simulink library "xrbsDSP_r4"  (Simulink 7.1)
undefined symbols (not defined in the file or in its folder): mem
libraries: xbsIndex_r4 x330
(part 1 of 5)
settings Model: Creator=singhj  LastModifiedBy=sysgengroup

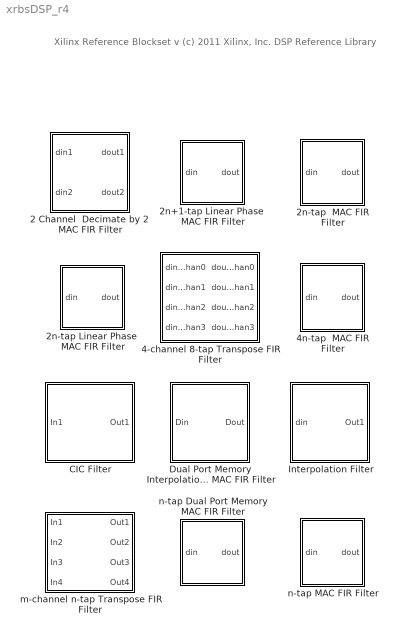
== system xrbsDSP_r4 ==
  note: Xilinx Reference Blockset v
      | (c) 2011 Xilinx, Inc.
      |
      | DSP Reference Library
  2 Channel  Decimate by 2  MAC FIR Filter : Subsystem  mask(n tap 2 Channel Decimate by 2 MAC FIR Filter){bit_width=18, bin_pt=16, coef1=fir1(60,.1), coef2=fir1(60,.3), coef_bit_width=18, coef_bin_pt=18, Ts=1}
      mask prompts: bit_width "Data Input Bit Width"; bin_pt "Data Input Binary Point"; coef1 "Coefficient Vector (Ch.1)"; coef2 "Coefficient Vector (Ch.2)"; coef_bit_width "Number of Bits per Coefficient"; coef_bin_pt "Binary Point per Coefficient"; Ts "Sample Period"
      mask help:
      | This is a n tap 2 Channel Filter decimate by 2 MAC Based FIR Filter.
      |
      |  - The Data Input bit width should be the same for both ports.
      |  - The number of Coefficients must be the same for both channels.
      |  - Pad coefficients with zeros if necessary.
      mask init:
      | %make sure there are an even number of coefficients
      | even_test1 = length(coef1)/2 - floor(length(coef1)/2);
      | if (even_test1 > 0)
      | 	coef1 = [coef1(:)' 0];
      | end
      | 
      | even_test2 = length(coef2)/2 - floor(length(coef2)/2);
      | if (even_test2 > 0)
      | 	coef2 = [coef2(:)' 0];
      | end
      | 
      | coef = 0;
      | j = 0;
      | 
      | for i = 1:2:length(coef1)
      | 
      | 	j = j+1;
      | 	coef(j) = coef1(i);
      | 
      | end
      | 
      | for i = 1:2:length(coef2)
      | 
      | 	j = j+1;
      | 	coef(j) = coef2(i);
      | 
      | end
      | 
      | for i = 2:2:length(coef1)
      | 
      | 	j = j+1;
      | 	coef(j) = coef1(i);
      | 
      | end
      | 
      | for i = 2:2:length(coef2)
      | 
      | 	j = j+1;
      | 	coef(j) = coef2(i);
      | 
      | end
      | 
      | %calculate the largest phase filter coefficient sum
      | 
      | %work in integers firstly
      | coef_int = coef*2^coef_bin_pt;
      | %Sum the coefficients
      | coef_sum1 = sum(abs(coef_int(1:length(coef_int)/4)));
      | coef_sum2 = sum(abs(coef_int(length(coef_int)/2+1:3*length(coef_int)/4)));
      | 
      | if coef_sum1 >= coef_sum2
      | 	coef_sum = coef_sum1;
      | else
      | 	coef_sum = coef_sum2;
      | end
      | 
      | %calculate the 2nd accumalator output width. Accomdates for poor coefficients
      | accum2_temp = ceil(log2(coef_sum*(2^(bit_width-1))))+1;
      | if accum2_temp < (bit_width+coef_bit_width)
      | 	accum2_bit_width = bit_width+coef_bit_width;
      | else
      | 	accum2_bit_width = accum2_temp;
      | end
      | 
      | %Graphic display
      | [bg,fg] = xlcmap('XBlock',0);
      | iPos = get_param(gcb,'Position');
      | iWidth=iPos(3)-iPos(1); iHeight=iPos(4)-iPos(2);
      | iCx=iWidth/2;
      | iCy=iHeight/2;
      | [logoX, logoY] = xlogo(iPos);
      mask Help: eval('');xlDoc('-book','sysgen','-topic','x2_Channel__Decimate_by_2__MAC_FIR_Filter');
      mask Display:
      | patch([0 iWidth iWidth 0],[0 0 iHeight iHeight] , bg);
      | patch(logoX,logoY , fg);
      | plot([0 0 iWidth iWidth 0], [0 iHeight iHeight 0 0]);
      | 
      | disp(sprintf('%d tap\nMAC FIR',length(coef)/2) )
      | 
      | port_label ('output',1,'yn0')
      | port_label ('output',2,'yn1')
      | port_label ('input',1,'xn0')
      | port_label ('input',2,'xn1')
  2n+1-tap Linear Phase  MAC FIR Filter : Subsystem  mask(2n+1-tap Linear Phase MAC FIR Filter){coef=fir1(32,.5), coef_n_bits=12, coef_bin_pt=11, smpl_n_bits=12, smpl_bin_pt=8, smpl_period=1}
      mask prompts: coef "Coefficients"; coef_n_bits "Number of Bits per Coefficient"; coef_bin_pt "Binary Point for Coefficient"; smpl_n_bits "Number of Bits per Input Sample"; smpl_bin_pt "Binary Point for Input Samples"; smpl_period "Input Sample Period"
      mask help: Linear phase MAC-based FIR filter with 2*n+1 coefficients. Design exploits odd coefficient symmetry.
      mask init:
      | dstr = sprintf('%d tap',length(coef));
      | 
      | [bg,fg] = xlcmap('XBlock',0);
      | iPos = get_param(gcb,'Position');
      | iWidth=iPos(3)-iPos(1); iHeight=iPos(4)-iPos(2);
      | iCx=iWidth/2;
      | iCy=iHeight/2;
      | [logoX, logoY] = xlogo(iPos);
      mask Help: eval('');xlDoc('-book','sysgen','-topic','x2n_1_tap_Linear_Phase__MAC_FIR_Filter');
      mask Display:
      | patch([0 iWidth iWidth 0],[0 0 iHeight iHeight] , bg);
      | patch(logoX,logoY, fg);
      | text(iCx/1.8,iCy+2,dstr);
      | text(iCx/2.0-4,iCy-10,'MAC FIR');
      | plot([0 0 iWidth iWidth 0], [0 iHeight iHeight 0 0]);
  2n-tap  MAC FIR Filter : Subsystem  mask(2n-tap MAC FIR Filter){coef=fir1(31,.5), coef_n_bits=12, coef_bin_pt=11, smpl_n_bits=12, smpl_bin_pt=8, smpl_period=1}
      mask prompts: coef "Coefficients"; coef_n_bits "Number of Bits per Coefficient"; coef_bin_pt "Binary Point for Coefficient"; smpl_n_bits "Number of Bits per Input Sample"; smpl_bin_pt "Binary Point for Input Samples"; smpl_period "Input Sample Period"
      mask help: MAC-based FIR filter with 2*n coefficients. Number of coefficients must be divisible by 2.
      mask init: same as xrbsDSP_r4/2n+1-tap Linear Phase  MAC FIR Filter
      mask Help: eval('');xlDoc('-book','sysgen','-topic','x2n_tap__MAC_FIR_Filter');
      mask Display:
      | patch([0 iWidth iWidth 0],[0 0 iHeight iHeight] , bg);
      | patch(logoX,logoY, fg);
      | text(iCx/1.8,iCy+2,dstr);
      | text(iCx/2.0-4,iCy-10,'MAC FIR');
      | plot([0 0 iWidth iWidth 0], [0 iHeight iHeight 0 0]);
  2n-tap Linear Phase  MAC FIR Filter : Subsystem  mask(2n-tap Linear Phase MAC FIR Filter){coef=fir1(31,.5), coef_n_bits=12, coef_bin_pt=11, smpl_n_bits=12, smpl_bin_pt=8, smpl_period=1}
      mask prompts: coef "Coefficients"; coef_n_bits "Number of Bits per Coefficient"; coef_bin_pt "Binary Point for Coefficient"; smpl_n_bits "Number of Bits per Input Sample"; smpl_bin_pt "Binary Point for Input Samples"; smpl_period "Input Sample Period"
      mask help: Linear phase MAC-based FIR filter with 2*n coefficients. Design exploits even coefficient symmetry.
      mask init: same as xrbsDSP_r4/2n+1-tap Linear Phase  MAC FIR Filter
      mask Help: eval('');xlDoc('-book','sysgen','-topic','x2n_tap_Linear_Phase__MAC_FIR_Filter');
      mask Display:
      | patch([0 iWidth iWidth 0],[0 0 iHeight iHeight] , bg);
      | patch(logoX,logoY, fg);
      | text(iCx/1.8,iCy+2,dstr);
      | text(iCx/2.0-4,iCy-10,'MAC FIR');
      | plot([0 0 iWidth iWidth 0], [0 iHeight iHeight 0 0]);
  4-channel 8-tap Transpose FIR Filter : Subsystem  mask(4-channel 8-tap Transpose FIR Filter){coef=fir1(7,.5), coef_n_bits=12, coef_bin_pt=11, smpl_n_bits=12, smpl_bin_pt=8, smpl_period=1}
      mask prompts: coef "Coefficients"; coef_n_bits "Number of Bits per Coefficient"; coef_bin_pt "Binary Point for Coefficient"; smpl_n_bits "Number of Bits per Input Sample"; smpl_bin_pt "Binary Point for Input Samples"; smpl_period "Input Sample Period"
      mask help: 4-channel 8-tap transpose FIR filter implemented using Virtex-II dedicated multipliers.
      mask init:
      | [bg,fg] = xlcmap('XBlock',0);
      | iPos = get_param(gcb,'Position');
      | iWidth=iPos(3)-iPos(1); iHeight=iPos(4)-iPos(2);
      | iCx=iWidth/2;
      | iCy=iHeight/2;
      | [logoX, logoY] = xlogo(iPos);
      mask Help: eval('');xlDoc('-book','sysgen','-topic','x4_channel_8_tap_Transpose_FIR_Filter');
      mask Display:
      | patch([0 iWidth iWidth 0],[0 0 iHeight iHeight] , bg);
      | patch(logoX,logoY, fg);
      | port_label('input',1,'xn0');
      | port_label('input',2,'xn1');
      | port_label('input',3,'xn2');
      | port_label('input',4,'xn3');
      | port_label('output',1,'yn0');
      | port_label('output',2,'yn1');
      | port_label('output',3,'yn2');
      | port_label('output',4,'yn3');
      | plot([0 0 iWidth iWidth 0], [0 iHeight iHeight 0 0]);
      | 
      | disp('8 Tap\n4 Channel\nTranspose\nFIR Filter')
  4n-tap  MAC FIR Filter : Subsystem  mask(4n-tap MAC FIR Filter){coef=fir1(63,.5), coef_n_bits=12, coef_bin_pt=11, smpl_n_bits=12, smpl_bin_pt=8, smpl_period=1}
      mask prompts: coef "Coefficients"; coef_n_bits "Number of Bits per Coefficient"; coef_bin_pt "Binary Point for Coefficient"; smpl_n_bits "Number of Bits per Input Sample"; smpl_bin_pt "Binary Point for Input Samples"; smpl_period "Input Sample Period"
      mask help: MAC-based FIR filter with 4*n coefficients. Number of coefficients must be divisible by 4.
      mask init:
      | dstr = sprintf('%d tap',length(coef));
      | 
      | [bg,fg] = xlcmap('XBlock',0);
      | iPos = get_param(gcb,'Position');
      | iWidth=iPos(3)-iPos(1); iHeight=iPos(4)-iPos(2);
      | iCx=iWidth/2;
      | iCy=iHeight/2;
      | [logoX, logoY] = xlogo(iPos);
      mask Help: eval('');xlDoc('-book','sysgen','-topic','x4n_tap__MAC_FIR_Filter');
      mask Display:
      | patch([0 iWidth iWidth 0],[0 0 iHeight iHeight] , bg);
      | patch(logoX,logoY, fg);
      | text(iCx/1.8,iCy+2,dstr);
      | text(iCx/2.0-4,iCy-10,'MAC FIR');
      | plot([0 0 iWidth iWidth 0], [0 iHeight iHeight 0 0]);
  CIC Filter : Subsystem  mask(CIC Filter){input_bitwidth=18, input_binpt=16, filter_type=Decimator, rate_change=48, stages=3, m=1, pipeline=on}
      mask prompts: input_bitwidth "Input Bit Width"; input_binpt "Input Binary Point"; filter_type "Filter Type"; rate_change "Sample Rate Change"; stages "Number of Stages"; m "Differential Delay"; pipeline "Pipeline Differentiators"
      mask help: Cascaded Integrated Comb (CIC) Filter
      mask init:
      | % CIC Single Channel v1.0
      | % Set Block Logo
      | sav_gcb=gcb;
      | [bg,fg] = xlcmap('XBlock',0);
      | iPos = get_param(sav_gcb,'Position');
      | iWidth=iPos(3)-iPos(1); iHeight=iPos(4)-iPos(2);
      | iCx=iWidth/2;
      | iCy=iHeight/2;
      | [logoX, logoY] = xlogo(iPos);
      | 
      | % Determine previous filter type and number of stages
      | prev_stages_list = find_system(sav_gcb, 'lookUnderMasks', 'all', 'FollowLinks', 'on', 'Regexp', 'on', 'Name', '^Integrator*'); %this is a cell array
      | prev_stages = length(prev_stages_list);
      | 
      | prev_filter_list = find_system(sav_gcb, 'lookUnderMasks', 'all', 'FollowLinks', 'on', 'Regexp', 'on', 'Name', '^Up Sample*'); %this is a cell array
      | if (isempty(prev_filter_list))
      |     prev_filter_list = find_system(sav_gcb, 'lookUnderMasks', 'all', 'FollowLinks', 'on', 'Regexp', 'on', 'Name', '^Down Sample*'); %this is a cell array
      |     if (isempty(prev_filter_list))
      |         errordlg('Previous Filter Type could not be determined')
      |     else
      |         prev_filter_type = 2;
      |     end
      | else
      |     prev_filter_type = 1;
      | end
      |   
      |   
      | % Print label on the block
      | if(filter_type == 2)
      |    cic_str = sprintf('%d-Stage\n CIC\n%d:1 Decimator',stages, rate_change);
      | else
      |    cic_str = sprintf('%d-Stage\n CIC\n1:%d Interpolator',stages, rate_change);	
      | end
      | 
      | % Make sure the entered values for stages and channels are positive integers
      | nstages = round(sum(abs(stages)));
      | 
      | % issue an error if the number of stages entered is zero
      | if (nstages == 0)
      | 	nstages = prev_stages;
      | 	errordlg('Number of Stages must be more than zero')
      | end
      | 
      | if (nstages == prev_stages) & (filter_type == prev_filter_type)
      |     return
      | end
      | 
      | if(filter_type == 2) % Decimator
      |    if (prev_filter_type == 1) % was interpolator so turn to decimator
      |        for i= 2:prev_stages,
      | 	      delete_line(sav_gcb, ['Integrator' int2str(i-1) '/' int2str(1)], ['Integrator' int2str(i) '/' int2str(1)]);
      | 	      delete_line(sav_gcb, ['Differentiator' int2str(i-1) '/' int2str(1)], ['Differentiator' int2str(i) '/' int2str(1)]);
      |        end
      | 
      |        % disconnect the last blocks in the two sections
      |        delete_line(sav_gcb, ['Differentiator' int2str(prev_stages) '/' int2str(1)], ['Up Sample/1']);
      |        delete_line(sav_gcb, ['Integrator' int2str(prev_stages) '/' int2str(1)], 'Out1/1');
      | 	
      | 	   % delete the line from the Up sampler to the Integrator
      | 	   delete_line(sav_gcb, 'Up Sample/1', 'Integrator1/1'); 
      | 	   delete_line(sav_gcb, 'In1/1', 'Differentiator1/1'); 
      | 	   
      | 	   % Delete the Up Sampler and then replace with an Down Sampler
      | 	   pup = get_param([sav_gcb '/Up Sample'], 'position');
      | 	   delete_block([sav_gcb '/Up Sample']);
      | 	   load_system('xbsIndex_r4');
      | 	   add_block('xbsIndex_r4/Down Sample', [sav_gcb '/Down Sample'], 'sample_ratio', 'rate_change','sample_phase', 'First Value of Frame', 'position', [pup(1), pup(2), pup(3),pup(4)]);
      | 	   
      | 	   % Switch the Integrators and Decimators around
      | 	   for i=1:prev_stages,
      | 		   tempi = get_param([sav_gcb '/Integrator' int2str(i)], 'position');
      | 	       tempd = get_param([sav_gcb '/Differentiator' int2str(i)], 'position');
      | 		   set_param([sav_gcb '/Differentiator' int2str(i)], 'position', [tempi(1), tempi(2), tempi(3), tempi(4)], 'output_bitwidth', 'ceil(stages*log2(rate_change*m) + input_bitwidth)');
      | 		   set_param([sav_gcb '/Integrator' int2str(i)], 'position', [tempd(1), tempd(2), tempd(3), tempd(4)]);
      | 	   end
      | 	   	   	
      | 	   % add back in the lines
      |        add_line(sav_gcb, 'In1/1', 'Integrator1/1', 'autorouting', 'on');
      | 	   add_line(sav_gcb, ['Integrator' int2str(prev_stages) '/1'], 'Down Sample/1', 'autorouting', 'on');
      | 	   add_line(sav_gcb, 'Down Sample/1', 'Differentiator1/1', 'autorouting', 'on');
      | 	   add_line(sav_gcb, ['Differentiator' int2str(prev_stages) '/1'], 'Out1/1', 'autorouting', 'on');
      | 	   for i= 2:prev_stages,
      |           add_line(sav_gcb, ['Integrator' int2str(i-1) '/1'], ['Integrator' int2str(i) '/' int2str(1)], 'autorouting', 'on');
      |           add_line(sav_gcb, ['Differentiator' int2str(i-1) '/1'], ['Differentiator' int2str(i) '/' int2str(1)], 'autorouting', 'on');
      | 	   end
      | 		
      |        %Set the Output bit widths of Differentiator and Integrator stages
      |        set_param([sav_gcb '/Differentiator1'], 'output_bitwidth', 'ceil(stages*log2(rate_change*m) + input_bitwidth)');
      | 	   	   %Set the Output bit width of Integrator stages
      | 	   %Calculate the Interpolator Integrator Output Bit Growth
      |        for i= 1:prev_stages,
      | 			 j = nstages+i;
      | 	         set_param([sav_gcb '/Integrator' int2str(i)], 'output_bitwidth', 'ceil(stages*log2(rate_change*m) + input_bitwidth)');
      |              set_param([sav_gcb '/Differentiator' int2str(i)], 'output_bitwidth', 'ceil(stages*log2(rate_change*m) + input_bitwidth)');
      | 	   end
      | 	   
      |    end
      |    
      |    if (nstages ~= prev_stages)
      |     
      |        % disconnect all the wires from all the blocks
      |        for i= 2:prev_stages,
      | 	      delete_line(sav_gcb, ['Integrator' int2str(i-1) '/' int2str(1)], ['Integrator' int2str(i) '/' int2str(1)]);
      | 	      delete_line(sav_gcb, ['Differentiator' int2str(i-1) '/' int2str(1)], ['Differentiator' int2str(i) '/' int2str(1)]);
      |        end
      | 
      |        % disconnect the last blocks in the two sections
      |        delete_line(sav_gcb, ['Integrator' int2str(prev_stages) '/' int2str(1)], ['Down Sample/1']);
      |        delete_line(sav_gcb, ['Differentiator' int2str(prev_stages) '/' int2str(1)], 'Out1/1');
      | 	
      | 	   % delete the line from the down sampler to the differentiator
      | 	   delete_line(sav_gcb, 'Down Sample/1', 'Differentiator1/1');
      | 	
      | 	   % Remove all the blocks except the first one (as we always will have one)
      |        for i=2:prev_stages,
      | 		  delete_block([sav_gcb '/Differentiator' int2str(i)]);
      | 	      delete_block([sav_gcb '/Integrator' int2str(i)]);
      |        end
      | 	   
      | 	   %Set the Output bit width of Differentiator stages
      |        set_param([sav_gcb '/Differentiator1'], 'output_bitwidth', 'ceil(stages*log2(rate_change*m) + input_bitwidth)');
      | 	   
      | 	   % collect data on the position of existing blocks
      | 	   pi = get_param([sav_gcb '/Integrator1'], 'position');
      | 	   pd = get_param([sav_gcb '/Differentiator1'], 'position');
      | 	   set_param([sav_gcb '/Differentiator1'], 'position', [pi(1)+(nstages+1)*80, pd(2), pi(3)+(nstages+1)*80, pd(4)]);
      | 	   pd = get_param([sav_gcb '/Differentiator1'], 'position');
      | 	
      | 	   % move the current blocks to accomadate for new blocks to be added 
      | 	   pds = get_param([sav_gcb '/Down Sample'], 'position');
      | 	   set_param([sav_gcb '/Down Sample'], 'position', [pi(1)+(nstages)*80, pds(2), pi(3)+(nstages)*80, pds(4)]);
      | 	   
      | 	   po = get_param([sav_gcb '/Out1'], 'position');
      | 	   set_param([sav_gcb '/Out1'], 'position', [pd(1)+(nstages+1)*80, po(2), pd(1)+(po(3)-po(1))+(nstages+1)*80, po(4)]);	
      | 	
      | 	   % add back in the line between the Down Sampler and the 1st Differentiator
      |        add_line(sav_gcb, 'Down Sample/1', ['Differentiator1/' int2str(1)], 'autorouting', 'on');
      | 
      | 	   % Only add blocks if more than one stage is required
      | 	   if (nstages ~= 1)
      | 		
      | 	       % Add in a copy of the first block to make up the required number of stages
      |            for i=2:nstages,
      |                add_block([sav_gcb '/Integrator1'], [sav_gcb '/Integrator' int2str(i)], 'position', [pi(1)+(i-1)*80, pi(2), pi(3)+(i-1)*80, pi(4)]);
      | 		       add_block([sav_gcb '/Differentiator1'], [sav_gcb '/Differentiator' int2str(i)], 'position', [pd(1)+(i-1)*80, pd(2), pd(3)+(i-1)*80, pd(4)]);
      | 	       end
      | 		
      | 	       % Connect up the wires to each block use autorouting
      |            for i= 2:nstages,
      |  		       add_line(sav_gcb, ['Integrator' int2str(i-1) '/' int2str(1)], ['Integrator' int2str(i) '/' int2str(1)], 'autorouting', 'on');
      | 	           add_line(sav_gcb, ['Differentiator' int2str(i-1) '/' int2str(1)], ['Differentiator' int2str(i) '/' int2str(1)], 'autorouting', 'on');
      |            end
      | 	    end
      | 	       % Connect the last blocks in the two sections
      |            add_line(sav_gcb, ['Integrator' int2str(nstages) '/' int2str(1)], ['Down Sample/1'], 'autorouting', 'on');
      |            add_line(sav_gcb, ['Differentiator' int2str(nstages) '/' int2str(1)], ['Out1/1'], 'autorouting', 'on');
      |    end
      | 
      | else % Interpolator
      |    
      | 	
      | 	if (prev_filter_type == 2) % was decimator so turn to interpolator
      | 	
      | 	  % disconnect all the wires from all the blocks
      |        for i= 2:prev_stages,
      | 	      delete_line(sav_gcb, ['Integrator' int2str(i-1) '/' int2str(1)], ['Integrator' int2str(i) '/' int2str(1)]);
      | 	      delete_line(sav_gcb, ['Differentiator' int2str(i-1) '/' int2str(1)], ['Differentiator' int2str(i) '/' int2str(1)]);
      |        end
      | 
      |        % disconnect the last blocks in the two sections
      |        delete_line(sav_gcb, ['Integrator' int2str(prev_stages) '/' int2str(1)], ['Down Sample/1']);
      |        delete_line(sav_gcb, ['Differentiator' int2str(prev_stages) '/' int2str(1)], 'Out1/1');
      | 	
      | 	   % delete the line from the down sampler to the Differentiator
      | 	   delete_line(sav_gcb, 'Down Sample/1', 'Differentiator1/1'); 
      | 	   delete_line(sav_gcb, 'In1/1', 'Integrator1/1'); 
      | 	   
      | 	   % Delete the Down Sampler and then replace with a Up Sampler
      | 	   pdwn = get_param([sav_gcb '/Down Sample'], 'position');
      | 	   delete_block([sav_gcb '/Down Sample']);
      | 	   load_system('xbsIndex_r4');
      | 	   add_block('xbsIndex_r4/Up Sample', [sav_gcb '/Up Sample'], 'sample_ratio', 'rate_change', 'position', [pdwn(1), pdwn(2), pdwn(3), pdwn(4)]);
      | 	   
      | 	   % Switch the Integrators and Decimators around
      | 	   for i=1:prev_stages,
      | 		   tempi = get_param([sav_gcb '/Integrator' int2str(i)], 'position');
      | 	       tempd = get_param([sav_gcb '/Differentiator' int2str(i)], 'position');
      | 		   set_param([sav_gcb '/Differentiator' int2str(i)], 'position', [tempi(1), tempi(2), tempi(3), tempi(4)], 'output_bitwidth', [int2str(i) '+ input_bitwidth']);
      | 		   set_param([sav_gcb '/Integrator' int2str(i)], 'position', [tempd(1), tempd(2), tempd(3), tempd(4)]);
      | 	   end
      | 	   	   	
      | 	   % add back in the lines
      |        add_line(sav_gcb, 'In1/1', 'Differentiator1/1', 'autorouting', 'on');
      | 	   add_line(sav_gcb, ['Differentiator' int2str(prev_stages) '/1'], 'Up Sample/1', 'autorouting', 'on');
      | 	   add_line(sav_gcb, 'Up Sample/1', 'Integrator1/1', 'autorouting', 'on');
      | 	   add_line(sav_gcb, ['Integrator' int2str(prev_stages) '/1'], 'Out1/1', 'autorouting', 'on');
      | 	   for i= 2:prev_stages,
      |           add_line(sav_gcb, ['Integrator' int2str(i-1) '/1'], ['Integrator' int2str(i) '/1'], 'autorouting', 'on');
      |           add_line(sav_gcb, ['Differentiator' int2str(i-1) '/1'], ['Differentiator' int2str(i) '/1'], 'autorouting', 'on');
      | 	   end
      | 	   
      | 	   %Set the Output bit width of Integrator stages
      | 	   %Calculate the Interpolator Integrator Output Bit Growth
      |        for i= 1:prev_stages,
      | 			 j = nstages+i;
      | 	         set_param([sav_gcb '/Integrator' int2str(i)], 'output_bitwidth', ['ceil(log2(2^(2*stages-' int2str(j) ')*(rate_change*m)^(' int2str(j) '-stages)) + input_bitwidth)']);
      | 	   end
      | 		
      |    end
      |    
      | 	
      | 	if (nstages ~= prev_stages)
      |     
      |        % disconnect all the wires from all the blocks
      |        for i= 2:prev_stages,
      | 	      delete_line(sav_gcb, ['Integrator' int2str(i-1) '/' int2str(1)], ['Integrator' int2str(i) '/' int2str(1)]);
      | 	      delete_line(sav_gcb, ['Differentiator' int2str(i-1) '/' int2str(1)], ['Differentiator' int2str(i) '/' int2str(1)]);
      |        end
      | 
      |        % disconnect the last blocks in the two sections
      |        delete_line(sav_gcb, ['Differentiator' int2str(prev_stages) '/' int2str(1)], ['Up Sample/1']);
      |        delete_line(sav_gcb, ['Integrator' int2str(prev_stages) '/' int2str(1)], 'Out1/1');
      |        
      | 	
      | 	   % delete the line from the Up sampler to the Integrator1 for movement later
      | 	   delete_line(sav_gcb, 'Up Sample/1', 'Integrator1/1'); 
      | 	
      | 	   % Remove all the blocks except the first one (as we always will have one)
      |        for i=2:prev_stages,
      | 		  delete_block([sav_gcb '/Differentiator' int2str(i)]);
      | 	      delete_block([sav_gcb '/Integrator' int2str(i)]);
      |        end
      | 	
      | 	   %Set the Output bit width of first Differentiator stage (other are set as copies of this block)
      |        set_param([sav_gcb '/Differentiator1'], 'output_bitwidth', '1 + input_bitwidth');
      | 	   
      | 	   % collect data on the position of existing blocks
      | 	   pi = get_param([sav_gcb '/Integrator1'], 'position');
      | 	   pd = get_param([sav_gcb '/Differentiator1'], 'position');
      | 	   set_param([sav_gcb '/Integrator1'], 'position', [pd(1)+(nstages+1)*80, pi(2), pd(3)+(nstages+1)*80, pi(4)]);
      | 	   pi = get_param([sav_gcb '/Integrator1'], 'position');
      | 	
      | 	   % move the current blocks to accomadate for new blocks to be added 
      | 	   pus = get_param([sav_gcb '/Up Sample'], 'position');
      | 	   set_param([sav_gcb '/Up Sample'], 'position', [pd(1)+(nstages)*80, pus(2), pd(3)+(nstages)*80, pus(4)]);
      | 	
      | 	   po = get_param([sav_gcb '/Out1'], 'position');
      |        set_param([sav_gcb '/Out1'], 'position', [pi(1)+(nstages+1)*80, po(2), pi(1)+(po(3)-po(1))+(nstages+1)*80, po(4)]);	
      |       
      | 	
      | 	   % add back in the line between the Up Sampler and the 1st Integrator1
      | 	   add_line(sav_gcb, 'Up Sample/1', 'Integrator1/1', 'autorouting', 'on');
      | 	   
      | 	   % Only add blocks if more than one stage is required
      | 	   if (nstages ~= 1)
      | 		
      | 	       % Add in a copy of the first block to make up the required number of stages
      |            for i=2:nstages,
      |                add_block([sav_gcb '/Integrator1'], [sav_gcb '/Integrator' int2str(i)], 'position', [pi(1)+(i-1)*80, pi(2), pi(3)+(i-1)*80, pi(4)]);
      | 		       add_block([sav_gcb '/Differentiator1'], [sav_gcb '/Differentiator' int2str(i)], 'position', [pd(1)+(i-1)*80, pd(2), pd(3)+(i-1)*80, pd(4)], 'output_bitwidth', [int2str(i) '+ input_bitwidth']);
      | 	       end
      | 		
      | 	       % Connect up the wires to each block use autorouting
      |            for i= 2:nstages,
      |  		       add_line(sav_gcb, ['Integrator' int2str(i-1) '/' int2str(1)], ['Integrator' int2str(i) '/' int2str(1)], 'autorouting', 'on');
      | 	           add_line(sav_gcb, ['Differentiator' int2str(i-1) '/' int2str(1)], ['Differentiator' int2str(i) '/' int2str(1)], 'autorouting', 'on');
      |            end
      | 	    end
      | 	       % Connect the last blocks in the two sections
      |            add_line(sav_gcb, ['Differentiator' int2str(nstages) '/1'], ['Up Sample/1'], 'autorouting', 'on');
      |            add_line(sav_gcb, ['Integrator' int2str(nstages) '/1'], ['Out1/1'], 'autorouting', 'on');
      | 		   
      | 	     %Set the Output bit width of Integrator stages
      | 	     %Calculate the Interpolator Integrator Output Bit Growth
      |           for i= 1:nstages,
      | 			 j = nstages+i;
      | 	         set_param([sav_gcb '/Integrator' int2str(i)], 'output_bitwidth', ['ceil(log2(2^(2*stages-' int2str(j) ')*(rate_change*m)^(' int2str(j) '-stages)) + input_bitwidth)']);
      | 	      end
      |    end
      | 	  
      | end
      | 
      | 
      | % Set the pipelining to ON or OFF on the differentiators
      | if (pipeline == 0)
      | 	for i= 1:nstages
      | 		set_param([sav_gcb '/Differentiator' int2str(i), '/AddSub'], 'latency', '0')
      | 	end
      | else
      | 	for i= 1:nstages
      | 		set_param([sav_gcb '/Differentiator' int2str(i), '/AddSub'], 'latency' ,'1')
      | 	end
      | end
      settings: CopyFcn=set_param(gcb, 'MaskSelfModifiable', 'on', 'LinkStatus', 'none');
      mask Help: eval('');xlDoc('-book','sysgen','-topic','CIC_Filter');
      mask StyleString: edit,edit,popup(Interpolator|Decimator),edit,edit,popup(1|2|3|4),checkbox
      mask Display:
      | patch([0 iWidth iWidth 0],[0 0 iHeight iHeight] , bg);
      | patch(logoX,logoY , fg);
      | plot([0 0 iWidth iWidth 0], [0 iHeight iHeight 0 0]);
      | disp(cic_str)
  Dual Port Memory Interpolation MAC FIR Filter : Subsystem  mask(n-tap Interpolate by N Dual Port Block RAM MAC FIR filter ){bit_width=16, bin_pt=13, coef_raw=fir1(55,0.3), coef_bit_width=18, coef_bin_pt=17, interpolation_rate=1:4, Ts=1}
      mask prompts: bit_width "Data Input Bit Width"; bin_pt "Data input Binary Point"; coef_raw "Coefficients"; coef_bit_width "Number of Bits per Coefficient"; coef_bin_pt "Binary Point Per Coefficient"; interpolation_rate "Interpolation Ratio"; Ts "Sample Period"
      mask help: n-tap Interpolate by N Dual Port Block RAM MAC FIR filter
      mask init:
      | % Interpolation by N Filter v1.0 - 8/9/03
      | %adjust the Interpolation Parameter to give the correct value
      | ir = interpolation_rate + 1;
      | 
      | %calculate how many padding bits are required for BRAM storage
      | if ((coef_bit_width - bit_width)  < 0 )
      | 	data_pad_bits = 0;
      | 	coef_pad_bits = bit_width - coef_bit_width;
      | else
      | 	data_pad_bits = coef_bit_width - bit_width;
      | 	coef_pad_bits = 0;
      | end
      | 
      | %prepare the coefficients for Polyphase structure
      | 
      | no_mults = 1; % for this implementation
      | 
      | %pad the coefficients to be a multiple of the interp_ratio*no_mults
      | multiple_test = round(((ceil(length(coef_raw)/(ir*no_mults))) - (length(coef_raw)/(ir*no_mults))) * (ir*no_mults));
      | if (multiple_test > 0)
      | 	coef_raw = [coef_raw(:)' zeros(1,multiple_test)];
      | end
      | 
      | no_taps = length(coef_raw);
      | phase_taps_per_mult = no_taps/no_mults/ir;
      |     
      | %form phase filters
      | h = zeros(1, no_taps/ir);
      | for p = 0:(ir-1)
      |      h(p+1,:) = coef_raw(p+1: ir :(no_taps-ir+p+1));
      | end
      | 
      | %put the phase filters into one memory
      | coef = h(1,:);
      | for p = 2:ir
      | 	coef = [coef h(p,:)];
      | end
      | 
      | %work in integers firstly
      | coef_int = coef*2^coef_bin_pt;
      | %Sum the coefficients
      | coef_sum = sum(abs(coef_int(1:length(coef_int)/4)));
      | 
      | %calculate the accumalator output width. Accomdates for poor coefficients
      | accum_temp = ceil(log2(coef_sum*(2^(bit_width-1))))+1;
      | if accum_temp < (bit_width+coef_bit_width)
      | 	accum_bit_width = bit_width+coef_bit_width;
      | else
      | 	accum_bit_width = accum_temp;
      | end
      | 
      | dstr1 = sprintf('%d tap', no_taps);
      | dstr2 = sprintf('Interpolate');
      | dstr3 = sprintf('by %d', ir);
      | 
      | [bg,fg] = xlcmap('XBlock',0);
      | iPos = get_param(gcb,'Position');
      | iWidth=iPos(3)-iPos(1); iHeight=iPos(4)-iPos(2);
      | iCx=iWidth/2;
      | iCy=iHeight/2;
      | [logoX, logoY] = xlogo(iPos);
      mask Help: eval('');xlDoc('-book','sysgen','-topic','Dual_Port_Memory_Interpolation_MAC_FIR_Filter');
      mask StyleString: edit,edit,edit,edit,edit,popup(1:2|1:3|1:4|1:5|1:6|1:7|1:8|1:9|1:10),edit
      mask Display:
      | patch([0 iWidth iWidth 0],[0 0 iHeight iHeight] , bg);
      | patch(logoX,logoY, fg);
      | text(iCx/1.3,iCy+15,dstr1);
      | text(iCx/2,iCy+2,dstr2);
      | text(iCx/1.3,iCy-9,dstr3);
      | text(iCx/1.5-4,iCy-20,'MAC FIR');
      | plot([0 0 iWidth iWidth 0], [0 iHeight iHeight 0 0]);
  Interpolation Filter : Subsystem  mask(Interpolation Filter){bit_width=8, bin_pt=6, coef=fir1(28,0.3), coef_bit_width=14, coef_bin_pt=14, interp_rate=1:2, Ts=1}
      mask prompts: bit_width "Input Data Bit Width"; bin_pt "Input Data Binary Point"; coef "Coefficients"; coef_bit_width "Number of bits per Coefficient"; coef_bin_pt "Binary Point per Coefficient"; interp_rate "Interpolation Factor"; Ts "Sample Period"
      mask help:
      | n - tap Interpolation MAC FIR filter.
      |
      |  - Support Interpolation rates of 2, 4, and 8.
      |  - 4 Multiplier and 4 Block RAM Architecture
      |  - Slice estimate provided
      |
      | NOTE: The number of coefficients must be divisible by (4*interpolation factor). If not zeros are padded to the coefficients to insure they are.
      |
      | Hardware notes:
      | This filter employs a 4 multiplier architecture to compute the filter. The highest supported sample rate is calculated by the
      | (input sample rate*(number of cofficients/4))
      mask init:
      | %accounts for the pull down GUI value
      | if (interp_rate == 1)
      | 	interp_ratio = 2;
      | elseif (interp_rate == 2)
      | 	interp_ratio = 4;
      | elseif (interp_rate == 3) 	
      | 	interp_ratio = 8;
      | else 	
      | 	interp_ratio = 16;	
      | end
      | 
      | no_mults = 4; % for this implementation
      | 
      | %pad the coefficients to be a multiple of the interp_ratio*no_mults
      | multiple_test = ((ceil(length(coef)/(interp_ratio*no_mults))) - (length(coef)/(interp_ratio*no_mults))) * (interp_ratio*no_mults);
      | if (multiple_test > 0)
      | 	coef = [coef(:)' zeros(1,multiple_test)];
      | end
      | 
      | no_taps = length(coef);
      | phase_taps_per_mult = no_taps/no_mults/interp_ratio;
      |     
      | %form phase filters h(0:3,)
      | h = zeros(1, no_taps/interp_ratio);
      | for p = 0:(interp_ratio-1)
      |      h(p+1,:) = coef(p+1: interp_ratio :(no_taps-interp_ratio+p+1));
      | end
      | 
      | %form DRAM values
      | mem_space = interp_ratio*no_mults*2^(ceil(log2(no_taps/interp_ratio/no_mults)));
      |         
      | z = zeros(1,(mem_space-no_taps)/interp_ratio/no_mults);
      | %mem = zeros(no_mults,(mem_space/no_mults));
      | 
      | for m = 0:(no_mults-1)
      |     for p = 0:(interp_ratio-1)
      | 		i = p*(mem_space/no_mults/interp_ratio)+1:(p+1)*(mem_space/no_mults/interp_ratio);
      |         mem(m+1,i) = [h(p+1,(m*phase_taps_per_mult)+(1:phase_taps_per_mult)), z];
      |     end
      | end
      | 
      | no_phases = interp_ratio;
      | no_phase_taps = no_taps/no_phases;
      | x_SRL_depth = no_phase_taps/no_mults;
      | upsamp_by = x_SRL_depth*no_phases;
      | downsamp_by = upsamp_by/interp_ratio;
      | T_clock = Ts/upsamp_by;
      | bit_growth = 2 + ceil(log2(x_SRL_depth));
      | y_bit_width = bit_width + coef_bit_width + bit_growth;
      | 
      | %slice count calculation
      | % control module
      |     k = ceil(ceil(log2(x_SRL_depth))/2);
      |     p = ceil(ceil(log2(interp_ratio))/2);
      |     k_p_logic = ceil(ceil((2*k + 2*p)/4)/2); %approx # of LUTs
      |     
      |     % synch delay
      |     delay = ceil(ceil(5/16)/2);
      |     
      |     % h DRAM cost
      | 	h = ceil(4*length(mem(1,:))/16/2*coef_bit_width); % for distmem
      |  	h = 0;   %for BRAM
      | 
      | 	% x buffer
      |     x = ceil(4*ceil(x_SRL_depth/16)*bit_width/2);
      |     
      |     % adder tree
      |     stage1 = 2*ceil((bit_width+coef_bit_width+1)/2);
      |     stage2 = ceil((bit_width+coef_bit_width+2)/2);
      |     
      |     % acc stage
      |     acc = ceil(y_bit_width/2);
      |     capture = acc;
      |     
      |     % downsampling
      |     downsample = ceil(y_bit_width/2);
      | 
      | %Display graphic on the block
      | dstr1 = sprintf('%d tap', no_taps);
      | dstr2 = sprintf('Interpolate');
      | dstr3 = sprintf('by %d', interp_ratio);
      | 
      | [bg,fg] = xlcmap('XBlock',0);
      | iPos = get_param(gcb,'Position');
      | iWidth=iPos(3)-iPos(1); iHeight=iPos(4)-iPos(2);
      | iCx=iWidth/2;
      | iCy=iHeight/2;
      | [logoX, logoY] = xlogo(iPos);
      mask Help: eval('');xlDoc('-book','sysgen','-topic','Interpolation_Filter');
      mask StyleString: edit,edit,edit,edit,edit,popup(1:2|1:4|1:8|1:16),edit
      mask Display:
      | patch([0 iWidth iWidth 0],[0 0 iHeight iHeight] , bg);
      | patch(logoX,logoY, fg);
      | text(iCx/1.3,iCy+15,dstr1);
      | text(iCx/2,iCy+2,dstr2);
      | text(iCx/1.3,iCy-9,dstr3);
      | text(iCx/1.5-4,iCy-20,'MAC FIR');
      | plot([0 0 iWidth iWidth 0], [0 iHeight iHeight 0 0]);
  m-channel n-tap Transpose FIR Filter : Subsystem  mask(Transpose Multi Channel FIR Filter){input_bitwidth=12, input_binpt=10, coef_array=fliplr(fir1(13, 0.31)), coef_bitwidth=16, coef_binpt=14, channels=4, tdm_fe=on, tdd_be=on, Ts=1, area2=[0, 0, 0, 0, 0, 0, 0], use_area2=on, prev_ncoef=14, prev_input_channels=4, prev_output_channels=4}
      mask prompts: input_bitwidth "Input Bit Width"; input_binpt "Input Binary Point"; coef_array "Coefficients (specify in reverse order)"; coef_bitwidth "Coefficients Bit Width"; coef_binpt "Coefficients Binary Point"; channels "Number of Channels"; tdm_fe "Time Division Multiplexer Front End"; tdd_be "Time Division DeMultiplexer Back End"; Ts "Input Sample Period"; area2 "FPGA Area [Slices, FFs, BRAMs, LUTs, IOBs, Emb. Mults, TBUFs]"; use_area2 "Use Area Above For Estimation"; prev_ncoef "Previous Coeff Value"; prev_input_channels "Previous Input Channels"; prev_output_channels "Previous Output Channels"
      mask help:
      | This Parametric Multi-Channel Transpose FIR Filter uses a fully parallel architecture with Time Division Multiplexing. The Time Division Multiplexer and Time Division Demux can be selected to be implemented or not. Embedded Multipliers are used for the multipliers.
      |
      | As the number of coefficients change so to does the structure underneath as the model is dynamically built.
      mask init:
      | sav_gcb=gcb;
      | sav_gcbh= gcbh;
      | % Set Block Logo
      | [bg,fg] = xlcmap('XBlock',0);
      | iPos = get_param(sav_gcb,'Position');
      | iWidth=iPos(3)-iPos(1); iHeight=iPos(4)-iPos(2);
      | iCx=iWidth/2;
      | iCy=iHeight/2;
      | [logoX, logoY] = xlogo(iPos);	
      | 
      | % Calculate Coefficient Specific Output Bit Width
      | % Note:  As the input type is not known (signed or unsigned), the
      | % worst case is assumed; hence use of largest unsigned input value
      | % for the given input bitwidth below.
      | magnitudeLargestUnsignedInput = 2^(input_bitwidth);
      | scaledCoefArray = coef_array * (2^coef_binpt);
      | sumOfLargestProducts = sum(scaledCoefArray * magnitudeLargestUnsignedInput);
      | output_bitwidth = ceil(log2(sumOfLargestProducts)) + 1;  % Add one for sign bit.
      | 
      | output_binpt = input_binpt + coef_binpt;
      | if (output_binpt > output_bitwidth)
      | 	output_binpt = output_bitwidth;
      | end
      | 
      | % Print label on the block
      | str = sprintf('%d Tap\n%d Channel\nTranspose\n FIR Filter',length(coef_array), channels);
      | 
      | 
      | % Make sure the entered value for channels is positive integers
      | nchannels = round(sum(abs(channels)));
      | ncoef = length(coef_array);
      | 
      | % How many input or output channels are required
      | if (tdm_fe == 0)
      | 	input_channels = 1;
      | 	% The latency through the TDM block 
      | 	p = 0;
      | else
      | 	input_channels = nchannels;
      | 	% The latency through the TDM block 
      | 	p = 1;
      | end
      | 
      | if (tdd_be == 0)
      | 	output_channels = 1;
      | else
      | 	output_channels = nchannels;
      | end
      | 
      | % Required for naming the port labels. This section creates an array of names for the icon panel to put on the block
      | ports_in = [1:input_channels 1+zeros(1,256-input_channels)];
      | ports_out = [1:output_channels 1+zeros(1,256-output_channels)];
      | 
      | port_inputnames = cell(256, 1);
      | port_outputnames = cell(256, 1);
      | port_inputnames(:,:) = cellstr('xn0');
      | port_outputnames(:,:) = cellstr('yn0');
      | 
      | for i=1:input_channels,
      | 	port_inputnames(i) = cellstr(['xn' int2str(i-1)]);
      | end
      | for i=1:output_channels,
      | 	port_outputnames(i) = cellstr(['yn' int2str(i-1)]);
      | end
      | % Print label on the block
      | m_str = sprintf('%d Tap\n%d Channel\nTranspose\n FIR Filter',length(coef_array), channels);
      | 
      | % Calculate how many channels are currently in the model
      | % pci = find_system([sav_gcb '/TDM'], 'lookUnderMasks', 'all', 'FollowLinks','on','Blocktype', 'Inport'); %this is a cell array
      | % pco = find_system([sav_gcb '/TDD'], 'lookUnderMasks', 'all', 'FollowLinks','on','Blocktype', 'Outport'); %this is a cell array
      | % prev_input_channels = length(pci(:,1));
      | % prev_output_channels = length(pco(:,1));
      | % %calculate how many coefficients currently in the model
      | % c = find_system(sav_gcb, 'lookUnderMasks', 'all', 'FollowLinks','on','masktype', 'MAD Block');
      | % prev_ncoef = length(c(:,1));
      | 
      | %error check for less than two coefficients
      | if (ncoef < 2)
      | 	ncoef = prev_ncoef;
      | 	errordlg('Number of Coefficients must be at least two')
      | end
      | 
      | if (ncoef ~= prev_ncoef)
      |     
      |        % disconnect all the wires from all the blocks
      |        for i= 2:prev_ncoef,
      | 	      delete_line(sav_gcb, ['MAD' int2str(i-1) '/1'], ['MAD' int2str(i) '/2']);
      | 	      delete_line(sav_gcb, ['TDM/1'], ['MAD' int2str(i) '/1']);
      |        end
      | 
      |        % disconnect the last block
      |        delete_line(sav_gcb, ['MAD' int2str(prev_ncoef) '/1'], ['TDD/1']);
      |        for i=1:prev_output_channels,
      | 	       delete_line(sav_gcb, ['TDD/' int2str(i)], ['Out' int2str(i) '/1']); 
      | 	   end
      | 	   
      | 	   % Remove all the blocks except the first two (as we always will have two)
      |        for i=3:prev_ncoef,
      | 		  delete_block([sav_gcb '/MAD' int2str(i)]);
      |        end
      | 	
      | 	   % collect data on the position of existing blocks
      | 	   pmad = get_param([sav_gcb '/MAD2'], 'position');
      | 	 
      | 	   % move the current blocks to accomadate for new blocks to be added 
      | 	   for i=1:prev_output_channels,
      | 	      po = get_param([sav_gcb '/Out' int2str(i)], 'position');
      | 	      set_param([sav_gcb '/Out' int2str(i)], 'position', [pmad(1)+(ncoef)*80, po(2), pmad(1)+(po(3)-po(1))+(ncoef)*80, po(4)]);	
      |        end
      | 	   
      | 	   ptdd = get_param([sav_gcb '/TDD'], 'position');
      | 	   set_param([sav_gcb '/TDD'], 'position', [pmad(1)+(ncoef-1)*80, ptdd(2), pmad(1)+(ptdd(3)-ptdd(1))+(ncoef-1)*80, ptdd(4)]);
      | 	
      | 	   % Only add MAD blocks if more than two taps are required
      | 	   if (ncoef ~= 2)
      | 		
      | 	       % Add in a copy of the first MAD block to make up the required number of coef
      |            for i=3:ncoef,
      |                add_block([sav_gcb '/MAD1'], [sav_gcb '/MAD' int2str(i)], 'position', [pmad(1)+(i-2)*80, pmad(2), pmad(3)+(i-2)*80, pmad(4)], 'coef', ['coef_array(' int2str(i) ')'], 'channels', 'channels');
      | 		   end
      | 		
      | 	       % Connect up the wires to each block use autorouting
      |            for i= 2:ncoef,
      |  		       add_line(sav_gcb, ['MAD' int2str(i-1) '/1'], ['MAD' int2str(i) '/2'], 'autorouting', 'on');
      | 	           add_line(sav_gcb, 'TDM/1', ['MAD' int2str(i) '/1'], 'autorouting', 'on');
      |            end
      | 	   end
      | 	       % Connect the last blocks in the two sections
      |            add_line(sav_gcb, ['MAD' int2str(ncoef) '/1'], ['TDD/1'], 'autorouting', 'on');
      | 		   for i=1:prev_output_channels,
      | 		       add_line(sav_gcb, ['TDD/' int2str(i)], ['Out' int2str(i) '/1'], 'autorouting', 'on');  
      | 		   end
      | end
      | 
      | %%%%%%%%%%%%%%%%%%%%%%%%%%%%%%%%%%%%%%%%%%%%%%%%%%%%%%%%%%%%%%%%%%%%%%%%%%%%%%%%%%%%%%%%%%%%%%%%%%
      | % Rebuild the Time Division Multiplexer and capture registers for the required number of channels %
      | %%%%%%%%%%%%%%%%%%%%%%%%%%%%%%%%%%%%%%%%%%%%%%%%%%%%%%%%%%%%%%%%%%%%%%%%%%%%%%%%%%%%%%%%%%%%%%%%%%
      | 
      | % issue an error if the number of channels entered is zero
      | if (nchannels == 0)
      | 	input_channels = prev_input_channels;
      | 	output_channels = prev_output_channels;
      | 	errordlg('Number of Channels must be more that zero');
      | end
      | 
      | % INPUT CHANNEL BUILDER
      | if (input_channels ~= prev_input_channels)
      | 	%special case 1 channel as no TDM required
      | 	if(input_channels == 1)
      | 		% disconnect upper level blocks on TDM
      | 		for i= 2:prev_input_channels,
      | 	   	   delete_line(sav_gcb, ['In' int2str(i) '/1'], ['TDM/' int2str(i)]);
      | 	    end
      | 		
      | 		% Remove all the inports except the first one (as we always will have one)
      |         for i=2:prev_input_channels,
      | 		    delete_block([sav_gcb '/In' int2str(i)]);
      | 		end
      | 		
      | 		% disconnect all the wires from all the blocks in the TDM
      |     	delete_line([sav_gcb '/TDM'], 'Counter/1', 'Mux1/1');
      | 		delete_line([sav_gcb '/TDM'], 'Mux1/1', 'Out1/1');
      | 		
      | 		for i= 1:prev_input_channels,
      | 	   	   delete_line([sav_gcb '/TDM'], ['In' int2str(i) '/1'], ['Up Sample' int2str(i) '/1']);
      | 		   delete_line([sav_gcb '/TDM'], ['Up Sample' int2str(i) '/1'], ['Mux1/' int2str(i+1)]);
      | 	    end
      | 				
      | 		%delete all blocks as no TDM required
      |         for i=2:prev_input_channels,
      | 		   delete_block([sav_gcb '/TDM/In' int2str(i)]);
      |         end
      | 		
      | 		for i=1:prev_input_channels,
      | 		   delete_block([sav_gcb '/TDM/Up Sample' int2str(i)]);
      |         end
      | 		
      | 		delete_block([sav_gcb '/TDM/Counter']);
      | 		delete_block([sav_gcb '/TDM/Mux1']);
      | 		
      | 		add_line([sav_gcb '/TDM'], 'In1/1', 'Out1/1', 'autorouting', 'on');
      | 		
      | 		
      | 		
      |     else
      | 
      | 	  % Create the TDM system for the specified number of channels
      | 	    
      |         % get position information on the Inports on both levels of hierarchy to help arrange the other blocks
      | 	    pinp = get_param([sav_gcb '/TDM/In1'], 'position');	
      | 		pinp_top = get_param([sav_gcb '/In1'], 'position');	
      | 
      | 
      | 	    % Do the required blocks already exist?
      | 	    if(prev_input_channels ~= 1) % Yes they do
      | 
      |            prev_input_channels
      | 		   % disconnect all the wires from all Input Blocks to the Mux
      | 		   for i= 1:prev_input_channels,
      | 	   	      delete_line([sav_gcb '/TDM'], ['In' int2str(i) '/1'], ['Up Sample' int2str(i) '/1']);
      | 			  delete_line([sav_gcb '/TDM'], ['Up Sample' int2str(i) '/1'], ['Mux1/' int2str(i+1)]);
      |            end
      | 
      | 		   for i= 2:prev_input_channels,
      | 		      delete_line(sav_gcb, ['In' int2str(i) '/1'], ['TDM/' int2str(i)]);
      |            end
      | 		   % delete all the Inports except the first one
      | 		   for i= 2:prev_input_channels,
      | 	   	      delete_block([sav_gcb '/TDM/In' int2str(i)]); 
      | 			  delete_block([sav_gcb '/In' int2str(i)]);  
      | 			  delete_block([sav_gcb '/TDM/Up Sample' int2str(i)]);
      | 	       end
      | 		   
      | 	    else
      | 		
      | 		   delete_line([sav_gcb '/TDM'], 'In1/1', 'Out1/1');
      | 		   		   	
      | 		   % Add all the necessary blocks to the TDM from the Xilinx Bloset Library 
      | 		   add_block('xbsIndex_r4/Mux', [sav_gcb '/TDM/Mux1'], 'position', [pinp(1)+200, pinp(2)-25, pinp(1)+230, pinp(2)+(25*input_channels)], 'latency', '1');
      | 		   add_block('xbsIndex_r4/Counter', [sav_gcb '/TDM/Counter'], 'position', [50, 50, 100, 100	]);
      | 		   add_block('xbsIndex_r4/Up Sample', [sav_gcb '/TDM/Up Sample1'], 'position', [pinp(1)+75, pinp(2)-5, pinp(1)+100, pinp(4)], 'copy_samples', 'on',  'sample_ratio', 'channels');
      | 		  
      | 		   add_line([sav_gcb '/TDM'], 'Counter/1', 'Mux1/1', 'autorouting', 'on');
      | 		   add_line([sav_gcb '/TDM'], 'Mux1/1', 'Out1/1', 'autorouting', 'on');
      | 		   
      | 	    end   
      | 		   
      | 		% Set the number of inputs on the MUX
      | 		set_param([sav_gcb '/TDM/Mux1'], 'inputs', int2str(input_channels), 'position', [pinp(1)+200, pinp(2)-25, pinp(1)+230, pinp(2)+(25*input_channels)]);
      | 		
      | 		% Add in a copy of the Inport and multiple TDD to make the required number channels on both levels of hierarchy
      | 		for i=2:input_channels,
      |             add_block([sav_gcb '/TDM/In1'], [sav_gcb '/TDM/In' int2str(i)], 'position', [pinp(1), pinp(2)+(i-1)*30, pinp(3), pinp(4)+(i-1)*30]);
      | 			add_block([sav_gcb '/In1'], [sav_gcb '/In' int2str(i)], 'position', [pinp_top(1), pinp_top(2)+(i-1)*30, pinp_top(3), pinp_top(4)+(i-1)*30]);
      | 			add_block([sav_gcb '/TDM/Up Sample1'], [sav_gcb '/TDM/Up Sample' int2str(i)], 'position', [pinp(1)+75, (pinp(2)-5)+(i-1)*30, pinp(1)+100, pinp(4)+(i-1)*30]);
      | 		end
      | 				
      | 		% Connect up the wires to each block in both levels of hierarchy using autorouting
      |         for i= 1:input_channels,
      |  		    add_line([sav_gcb '/TDM'], ['In' int2str(i) '/1'], ['Up Sample' int2str(i) '/1'], 'autorouting', 'on');
      | 			add_line([sav_gcb '/TDM'], ['Up Sample' int2str(i) '/1'], ['Mux1/' int2str(i+1)], 'autorouting', 'on');
      | 		end
      | 		for i= 2:input_channels,
      | 			add_line(sav_gcb, ['In' int2str(i) '/1'], ['TDM/' int2str(i)], 'autorouting', 'on');	
      | 		end
      | 		
      | 		% Setup the Counter and Constant parameters
      | 		set_param([sav_gcb '/TDM/Counter'], 'cnt_to', int2str(input_channels-1), 'arith_type', 'Unsigned', 'n_bits', int2str(ceil(log2(input_channels))), 'period', ['Ts/' int2str(input_channels)]);
      | 	 			
      | 		% reshape the TDM Block	and the CIC block
      | 		ptdm = get_param([sav_gcb '/TDM'], 'position');
      | 		set_param([sav_gcb '/TDM'], 'position', [ptdm(1), 40, ptdm(3), 20+input_channels*30]);
      | 				
      | 	end
      | end
      | 
      | 
      | % OUTPUT CHANNEL BUILDER
      | if (output_channels ~= prev_output_channels)
      | 	%special case 1 channel as no TDM required
      | 	if(output_channels == 1)
      | 		
      | 		% disconnect upper level blocks on TDD
      | 		for i= 2:prev_output_channels,
      | 		   delete_line(sav_gcb, ['TDD/' int2str(i)], ['Out' int2str(i) '/1']);
      | 	    end
      | 		
      | 		% Remove all the outports except the first one (as we always will have one)
      |         for i=2:prev_output_channels,
      | 			delete_block([sav_gcb '/Out' int2str(i)]);
      | 		end
      | 		
      | 		% disconnect all the wires from all the blocks in the TDD
      | 		for i= 1:prev_output_channels,
      | 		   delete_line([sav_gcb '/TDD'], ['In1/1'], ['Register' int2str(i) '/1']);
      | 		   delete_line([sav_gcb '/TDD'], ['Counter/1'], ['Relational' int2str(i) '/1']);
      | 		   delete_line([sav_gcb '/TDD'], ['Constant' int2str(i) '/1'], ['Relational' int2str(i) '/2']);
      | 		   delete_line([sav_gcb '/TDD'], ['Relational' int2str(i) '/1'], ['Register' int2str(i) '/2']);
      | 		   delete_line([sav_gcb '/TDD'], ['Register' int2str(i) '/1'], ['Down Sample' int2str(i) '/1']);
      | 		   delete_line([sav_gcb '/TDD'], ['Down Sample' int2str(i) '/1'], ['Out' int2str(i) '/1']);
      | 	    end
      | 				
      | 		%delete all blocks as no TDD required
      |         for i=2:prev_output_channels,  	   
      | 		   delete_block([sav_gcb '/TDD/Out' int2str(i)]);  	  
      |         end
      | 		
      | 		for i=1:prev_output_channels,
      | 		   delete_block([sav_gcb '/TDD/Down Sample' int2str(i)]);  
      | 		   delete_block([sav_gcb '/TDD/Register' int2str(i)]);  	   
      | 		   delete_block([sav_gcb '/TDD/Constant' int2str(i)]); 
      | 		   delete_block([sav_gcb '/TDD/Relational' int2str(i)]);
      |         end
      | 	
      | 		delete_block([sav_gcb '/TDD/Counter']);
      | 		
      | 		add_line([sav_gcb '/TDD'], 'In1/1', 'Out1/1', 'autorouting', 'on');
      | 		
      | 		
      | 	else
      | 	
      | 	  % Create the TDD system for the specified number of channels
      | 	    
      |         % get position information on the Outports on both levels of hierarchy to help arrange the other blocks
      | 		pout = get_param([sav_gcb '/TDD/Out1'], 'position');	
      | 		pout_top = get_param([sav_gcb '/Out1'], 'position');	
      | 	
      | 	    % Do the required blocks already exist?
      | 	    if(prev_output_channels ~= 1) % Yes they do
      |  	       
      | 		   % disconnect all the wires from all the TDD Blocks
      | 		   for i= 1:prev_output_channels,
      | 			  delete_line([sav_gcb '/TDD'], ['In1/1'], ['Register' int2str(i) '/1']);
      | 		      delete_line([sav_gcb '/TDD'], ['Counter/1'], ['Relational' int2str(i) '/1']);
      | 		      delete_line([sav_gcb '/TDD'], ['Constant' int2str(i) '/1'], ['Relational' int2str(i) '/2']);   
      | 		      delete_line([sav_gcb '/TDD'], ['Relational' int2str(i) '/1'], ['Register' int2str(i) '/2']);
      | 		      delete_line([sav_gcb '/TDD'], ['Register' int2str(i) '/1'], ['Down Sample' int2str(i) '/1']);
      | 			  delete_line([sav_gcb '/TDD'], ['Down Sample' int2str(i) '/1'], ['Out' int2str(i) '/1']);
      | 		   end
      | 		   for i= 2:prev_output_channels,
      | 			  delete_line(sav_gcb, ['TDD/' int2str(i)], ['Out' int2str(i) '/1']);
      | 		   end
      | 		   
      | 		   % delete all the Inports and the main blocks of the TDD except the first one
      | 		   for i= 2:prev_output_channels,  
      | 			  delete_block([sav_gcb '/TDD/Out' int2str(i)]); 
      | 			  delete_block([sav_gcb '/Out' int2str(i)]); 
      | 			  delete_block([sav_gcb '/TDD/Down Sample' int2str(i)]);
      | 			  delete_block([sav_gcb '/TDD/Register' int2str(i)]);  	   
      | 		      delete_block([sav_gcb '/TDD/Constant' int2str(i)]); 
      | 		      delete_block([sav_gcb '/TDD/Relational' int2str(i)]);
      | 	       end
      | 		   
      | 	    else
      | 		
      | 		   delete_line([sav_gcb '/TDD'], 'In1/1', 'Out1/1');
      | 		   	
      | 		   % Add all the necessary blocks to TDD
      | 		   add_block('xbsIndex_r4/Counter', [sav_gcb '/TDD/Counter'], 'position', [70,   130,   120,   180]);
      | 		   add_block('xbsIndex_r4/Constant', [sav_gcb '/TDD/Constant1'], 'position', [205,   164,   220,   186]);
      | 		   add_block('xbsIndex_r4/Relational', [sav_gcb '/TDD/Relational1'], 'position', [245,   143,   290,   187]);
      | 		   add_block('xbsIndex_r4/Register', [sav_gcb '/TDD/Register1'], 'position', [395,    102,   440,   153]);
      | 		   add_block('xbsIndex_r4/Down Sample', [sav_gcb '/TDD/Down Sample1'], 'sample_ratio', 'channels', 'position', [495,    102,   540,   153]);
      | 		   
      | 		   set_param([sav_gcb '/TDD/Register1'], 'en', 'on');
      | 	 
      | 	    end   
      | 		  		
      | 		% Add in a copy of the multiple TDD to make the required number channels on both levels of hierarchy
      | 		for i=2:output_channels,
      |             add_block([sav_gcb '/TDD/Out1'], [sav_gcb '/TDD/Out' int2str(i)], 'position', [pout(1), pout(2)+(i-1)*75, pout(3), pout(4)+(i-1)*75]);
      | 			add_block([sav_gcb '/Out1'], [sav_gcb '/Out' int2str(i)], 'position', [pout_top(1), pout_top(2)+(i-1)*30, pout_top(3), pout_top(4)+(i-1)*30]);
      | 		    add_block([sav_gcb '/TDD/Constant1'], [sav_gcb '/TDD/Constant' int2str(i)], 'position', [205,   164+((i-1)*75),   220,   186+((i-1)*75)]);
      | 		    add_block([sav_gcb '/TDD/Relational1'], [sav_gcb '/TDD/Relational' int2str(i)], 'position', [245,   143+((i-1)*75),   290,   187+((i-1)*75)]);
      | 		    add_block([sav_gcb '/TDD/Register1'], [sav_gcb '/TDD/Register' int2str(i)], 'position', [395,    102+((i-1)*75),   440,   153+((i-1)*75)]);
      | 			add_block([sav_gcb '/TDD/Down Sample1'], [sav_gcb '/TDD/Down Sample' int2str(i)], 'position', [495,    102+((i-1)*75),   540,   153+((i-1)*75)]);
      | 		end
      | 				
      | 		% Connect up the wires to each block in both levels of hierarchy using autorouting
      |         for i= 1:output_channels,
      |  			add_line([sav_gcb '/TDD'], 'Counter/1', ['Relational' int2str(i) '/1'], 'autorouting', 'on');
      | 			add_line([sav_gcb '/TDD'], ['Constant' int2str(i) '/1'], ['Relational' int2str(i) '/2'], 'autorouting', 'on');
      | 			add_line([sav_gcb '/TDD'], ['Relational' int2str(i) '/1'], ['Register' int2str(i) '/2'], 'autorouting', 'on');
      | 			add_line([sav_gcb '/TDD'], 'In1/1', ['Register' int2str(i) '/1'], 'autorouting', 'on');
      | 			add_line([sav_gcb '/TDD'], ['Register' int2str(i) '/1'], ['Down Sample' int2str(i) '/1'], 'autorouting', 'on');
      | 			add_line([sav_gcb '/TDD'], ['Down Sample' int2str(i) '/1'], ['Out' int2str(i) '/1'], 'autorouting', 'on');
      | 		end
      | 		for i= 2:output_channels,
      | 		    add_line(sav_gcb, ['TDD/' int2str(i)], ['Out' int2str(i) '/1'], 'autorouting', 'on');
      | 		end
      | 
      | 		% Setup the TDD Counter and Constant parameters
      | 		if (nchannels > 1)
      | 			set_param([sav_gcb '/TDD/Counter'], 'cnt_to', int2str(nchannels-1), 'n_bits', 'ceil(log2(channels))', 'arith_type', 'Unsigned', 'n_bits', int2str(ceil(log2(output_channels))), 'period', ['Ts/' int2str(output_channels)]);
      | 		end
      | 		
      | 	    for i=1:output_channels,   
      | 			set_param([sav_gcb '/TDD/Constant' int2str(i)], 'const', int2str(i-1), 'arith_type', 'Unsigned', 'n_bits', int2str(ceil(log2(i+1))),'bin_pt','0');
      | 		end
      | 		
      | 		% reshape the TDD Block	and the CIC block
      | 		ptdd = get_param([sav_gcb '/TDD'], 'position');
      | 		set_param([sav_gcb '/TDD'], 'position', [ptdd(1), 40, ptdd(3), 20+output_channels*30]);
      | 		pcic = get_param(sav_gcb, 'position');
      | 		set_param(sav_gcb, 'position', [pcic(1), pcic(2), pcic(3), pcic(4)-(5*prev_output_channels)+(5*output_channels)]);
      | 				
      |     end
      |     % Calculate Latency through the filter and which channel comes out first
      |     L = 1 + (3 + (nchannels-1));
      | 	r = rem(L,nchannels);
      | 	co = [r:nchannels-1 0:r-1];
      | 	if (output_channels > 1)	
      |         for i=1:output_channels,
      |             set_param([sav_gcb '/TDD/Constant' int2str(i)], 'const', int2str(co(i)), 'arith_type', 'Unsigned', 'n_bits', int2str(ceil(log2(co(i)+2))));
      |         end
      |     end
      | end
      | 
      | % Set the overide with doubles on with selected
      | % Find all the Xilinx Blocks in the system
      | if (ncoef ~= prev_ncoef)
      |     set_param(sav_gcbh, 'prev_ncoef', int2str(ncoef));
      | end
      | 
      | if (input_channels ~= prev_input_channels)
      |     set_param(sav_gcbh, 'prev_input_channels', int2str(input_channels));
      | end
      | 
      | if (output_channels ~= prev_output_channels)
      |     set_param(sav_gcbh, 'prev_output_channels', int2str(output_channels));
      |     prev_output_channels = output_channels;
      | end
      settings: CopyFcn=set_param(gcb, 'MaskSelfModifiable', 'on', 'LinkStatus', 'none');
      mask Help: eval('');xlDoc('-book','sysgen','-topic','m_channel_n_tap_Transpose_FIR_Filter');
      mask Display:
      | patch([0 iWidth iWidth 0],[0 0 iHeight iHeight] , bg);
      | patch(logoX,logoY , fg);
      | plot([0 0 iWidth iWidth 0], [0 iHeight iHeight 0 0]);
      | port_label('input',ports_in(1), char(port_inputnames(1)))
      | port_label('input',ports_in(2), char(port_inputnames(2)))
      | port_label('input',ports_in(3), char(port_inputnames(3)))
      | port_label('input',ports_in(4), char(port_inputnames(4)))
      | port_label('input',ports_in(5), char(port_inputnames(5)))
      | port_label('input',ports_in(6), char(port_inputnames(6)))
      | port_label('input',ports_in(7), char(port_inputnames(7)))
      | port_label('input',ports_in(8), char(port_inputnames(8)))
      | port_label('input',ports_in(9), char(port_inputnames(9)))
      | port_label('input',ports_in(10), char(port_inputnames(10)))
      | port_label('input',ports_in(11), char(port_inputnames(11)))
      | port_label('input',ports_in(12), char(port_inputnames(12)))
      | port_label('input',ports_in(13), char(port_inputnames(13)))
      | port_label('input',ports_in(14), char(port_inputnames(14)))
      | port_label('input',ports_in(15), char(port_inputnames(15)))
      | port_label('input',ports_in(16), char(port_inputnames(16)))
      | port_label('input',ports_in(17), char(port_inputnames(17)))
      | port_label('input',ports_in(18), char(port_inputnames(18)))
      | port_label('input',ports_in(19), char(port_inputnames(19)))
      | port_label('input',ports_in(20), char(port_inputnames(20)))
      | port_label('input',ports_in(21), char(port_inputnames(21)))
      | port_label('input',ports_in(22), char(port_inputnames(22)))
      | port_label('input',ports_in(23), char(port_inputnames(23)))
      | port_label('input',ports_in(24), char(port_inputnames(24)))
      | port_label('input',ports_in(25), char(port_inputnames(25)))
      | port_label('input',ports_in(26), char(port_inputnames(26)))
      | port_label('input',ports_in(27), char(port_inputnames(27)))
      | port_label('input',ports_in(28), char(port_inputnames(28)))
      | port_label('input',ports_in(29), char(port_inputnames(29)))
      | port_label('input',ports_in(30), char(port_inputnames(30)))
      | port_label('input',ports_in(31), char(port_inputnames(31)))
      | port_label('input',ports_in(32), char(port_inputnames(32)))
      | port_label('output',ports_out(1), char(port_outputnames(1)))
      | port_label('output',ports_out(2), char(port_outputnames(2)))
      | port_label('output',ports_out(3), char(port_outputnames(3)))
      | port_label('output',ports_out(4), char(port_outputnames(4)))
      | port_label('output',ports_out(5), char(port_outputnames(5)))
      | port_label('output',ports_out(6), char(port_outputnames(6)))
      | port_label('output',ports_out(7), char(port_outputnames(7)))
      | port_label('output',ports_out(8), char(port_outputnames(8)))
      | port_label('output',ports_out(9), char(port_outputnames(9)))
      | port_label('output',ports_out(10), char(port_outputnames(10)))
      | port_label('output',ports_out(11), char(port_outputnames(11)))
      | port_label('output',ports_out(12), char(port_outputnames(12)))
      | port_label('output',ports_out(13), char(port_outputnames(13)))
      | port_label('output',ports_out(14), char(port_outputnames(14)))
      | port_label('output',ports_out(15), char(port_outputnames(15)))
      | port_label('output',ports_out(16), char(port_outputnames(16)))
      | port_label('output',ports_out(17), char(port_outputnames(17)))
      | port_label('output',ports_out(18), char(port_outputnames(18)))
      | port_label('output',ports_out(19), char(port_outputnames(19)))
      | port_label('output',ports_out(20), char(port_outputnames(20)))
      | port_label('output',ports_out(21), char(port_outputnames(21)))
      | port_label('output',ports_out(22), char(port_outputnames(22)))
      | port_label('output',ports_out(23), char(port_outputnames(23)))
      | port_label('output',ports_out(24), char(port_outputnames(24)))
      | port_label('output',ports_out(25), char(port_outputnames(25)))
      | port_label('output',ports_out(26), char(port_outputnames(26)))
      | port_label('output',ports_out(27), char(port_outputnames(27)))
      | port_label('output',ports_out(28), char(port_outputnames(28)))
      | port_label('output',ports_out(29), char(port_outputnames(29)))
      | port_label('output',ports_out(30), char(port_outputnames(30)))
      | port_label('output',ports_out(31), char(port_outputnames(31)))
      | port_label('output',ports_out(32), char(port_outputnames(32)))
      | disp(m_str)
  n-tap Dual Port Memory MAC FIR Filter : Subsystem  mask(n-tap Dual Port Block RAM MAC FIR filter ){bit_width=12, bin_pt=10, coef=fir1(159, 0.3), coef_bit_width=16, coef_bin_pt=16, Ts=1}
      mask prompts: bit_width "Data Input Bit Width"; bin_pt "Data input Binary Point"; coef "Coefficients"; coef_bit_width "Number of Bits per Coefficient"; coef_bin_pt "Binary Point Per Coefficient"; Ts "Sample Period"
      mask help: n-tap Single Rate Dual Port Block RAM MAC FIR filter
      mask init:
      | %calculate how many padding bits are required for BRAM storage
      | if ((coef_bit_width - bit_width)  < 0 )
      | 	data_pad_bits = 0;
      | 	coef_pad_bits = bit_width - coef_bit_width;
      | else
      | 	data_pad_bits = coef_bit_width - bit_width;
      | 	coef_pad_bits = 0;
      | end
      | 
      | %work in integers firstly
      | coef_int = coef*2^coef_bin_pt;
      | %Sum the coefficients
      | coef_sum = sum(abs(coef_int(1:length(coef_int)/4)));
      | 
      | %calculate the 2nd accumalator output width. Accomdates for poor coefficients
      | accum2_temp = ceil(log2(coef_sum*(2^(bit_width-1))))+1;
      | if accum2_temp < (bit_width+coef_bit_width)
      | 	accum_bit_width = bit_width+coef_bit_width;
      | else
      | 	accum_bit_width = accum2_temp;
      | end
      | 
      | dstr = sprintf('%d tap',length(coef));
      | 
      | [bg,fg] = xlcmap('XBlock',0);
      | iPos = get_param(gcb,'Position');
      | iWidth=iPos(3)-iPos(1); iHeight=iPos(4)-iPos(2);
      | iCx=iWidth/2;
      | iCy=iHeight/2;
      | [logoX, logoY] = xlogo(iPos);
      mask Help: eval('');xlDoc('-book','sysgen','-topic','n_tap_Dual_Port_Memory_MAC_FIR_Filter');
      mask Display:
      | patch([0 iWidth iWidth 0],[0 0 iHeight iHeight] , bg);
      | patch(logoX,logoY, fg);
      | text(iCx/2.1,iCy+6,dstr);
      | text(iCx/2.1-4,iCy-6,'MAC FIR');
      | plot([0 0 iWidth iWidth 0], [0 iHeight iHeight 0 0]);
  n-tap MAC FIR Filter : Subsystem  mask(n-tap MAC FIR Filter){coef=fir1(15,.5), coef_n_bits=12, coef_bin_pt=11, smpl_n_bits=12, smpl_bin_pt=8, smpl_period=1}
      mask prompts: coef "Coefficients"; coef_n_bits "Number of Bits per Coefficient"; coef_bin_pt "Binary Point for Coefficient"; smpl_n_bits "Number of Bits per Input Sample"; smpl_bin_pt "Binary Point for Input Samples"; smpl_period "Input Sample Period"
      mask help: MAC-based FIR filter with n coefficients.
      mask init: same as xrbsDSP_r4/2n+1-tap Linear Phase  MAC FIR Filter
      mask Help: eval('');xlDoc('-book','sysgen','-topic','n_tap_MAC_FIR_Filter');
      mask Display:
      | patch([0 iWidth iWidth 0],[0 0 iHeight iHeight] , bg);
      | patch(logoX,logoY, fg);
      | text(iCx/1.8,iCy+2,dstr);
      | text(iCx/2.0-4,iCy-10,'MAC FIR');
      | plot([0 0 iWidth iWidth 0], [0 iHeight iHeight 0 0]);
